simulink model "jacobianComparison"  (R2016a)
settings: Solver=ode4  StartTime=0.0  StopTime=10.0  FixedStep=0.001  RelTol=1e-3
libraries: lwr_dynamics x2
settings Model: Creator=shahriari  LastModifiedBy=shahriari

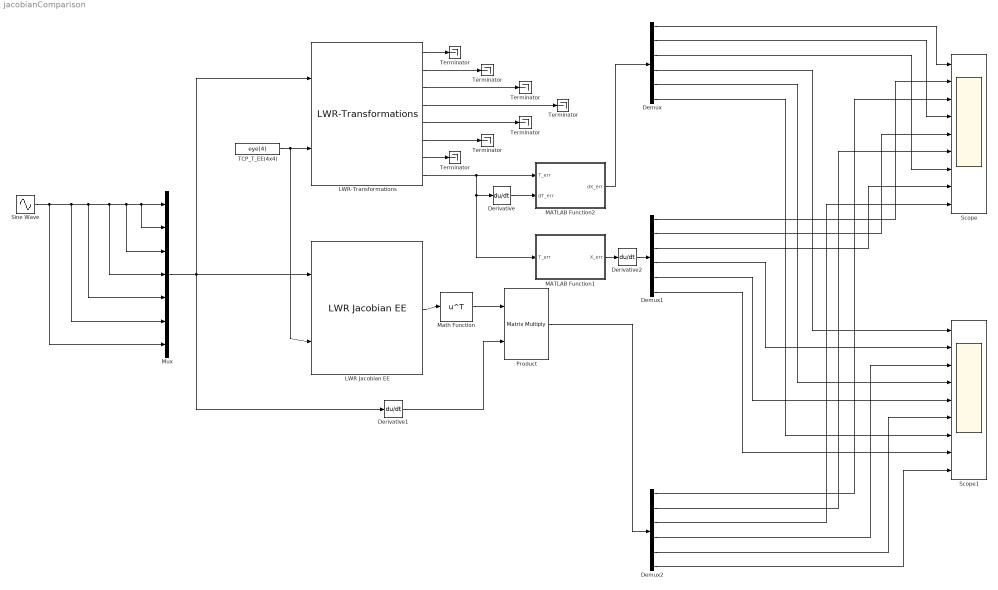
== system jacobianComparison ==
  Demux : Demux  Outputs=6
  Demux1 : Demux  Outputs=6
  Demux2 : Demux  Outputs=6
  Derivative : Derivative
  Derivative1 : Derivative
  Derivative2 : Derivative
  LWR Jacobian EE : lwr_dynamics/Kinematics/LWR Jacobian EE
  LWR-Transformations : lwr_dynamics/Kinematics/LWR-Transformations
  MATLAB Function1 : MATLAB Function  TreatAsAtomicUnit=on
  MATLAB Function2 : MATLAB Function  TreatAsAtomicUnit=on
  Math Function : Math  Operator=transpose  SaturateOnIntegerOverflow=on
  Mux : Mux  Inputs=7
  Product : Product  Multiplication=Matrix(*)
  Scope : Scope  NumInputPorts=9
  Scope1 : Scope  NumInputPorts=9
  Sine Wave : Sin  Bias=0.1  SampleTime=0
  TCP_T_EE(4x4) : Constant  Value=eye(4)
  Terminator : Terminator
  "Terminator " : Terminator
  "Terminator  " : Terminator
  "Terminator   " : Terminator
  "Terminator    " : Terminator
  "Terminator     " : Terminator
  "Terminator      " : Terminator
  wires:
  TCP_T_EE(4x4)/1 -> LWR Jacobian EE/2, LWR-Transformations/2
  Mux/1 -> LWR-Transformations/1, LWR Jacobian EE/1, Derivative1/1
  LWR-Transformations/1 -> Terminator/1
  LWR-Transformations/2 -> "Terminator "/1
  LWR-Transformations/3 -> "Terminator  "/1
  LWR-Transformations/4 -> "Terminator   "/1
  LWR-Transformations/5 -> "Terminator    "/1
  LWR-Transformations/6 -> "Terminator     "/1
  LWR-Transformations/7 -> "Terminator      "/1
  LWR Jacobian EE/1 -> Math Function/1
  Math Function/1 -> Product/1
  LWR-Transformations/8 -> MATLAB Function1/1(T_err), Derivative/1, MATLAB Function2/1(T_err)
  Derivative/1 -> MATLAB Function2/2(dT_err)
  Derivative1/1 -> Product/2
  MATLAB Function2/1(dX_err) -> Demux/1
  Product/1 -> Demux2/1
  MATLAB Function1/1(X_err) -> Derivative2/1
  Derivative2/1 -> Demux1/1
  Demux/1 -> Scope/1
  Demux/2 -> Scope/4
  Demux/3 -> Scope/7
  Demux1/1 -> Scope/2
  Demux1/2 -> Scope/5
  Demux1/3 -> Scope/8
  Demux2/1 -> Scope/3
  Demux2/2 -> Scope/6
  Demux2/3 -> Scope/9
  Demux/4 -> Scope1/1
  Demux/5 -> Scope1/4
  Demux/6 -> Scope1/7
  Demux1/4 -> Scope1/2
  Demux1/5 -> Scope1/5
  Demux1/6 -> Scope1/8
  Demux2/4 -> Scope1/3
  Demux2/5 -> Scope1/6
  Demux2/6 -> Scope1/9
  Sine Wave/1 -> Mux/7, Mux/6, Mux/5, Mux/4, Mux/3, Mux/2, Mux/1

== matlab function jacobianComparison/MATLAB Function1 ==
  data: T_err input; X_err output
function X_err  = fcn(T_err)
%#codegen

X_err = [T_err(1:3,4);rotm2eul(T_err(1:3,1:3))'];

== matlab function jacobianComparison/MATLAB Function2 ==
  data: T_err input; dX_err output; dT_err input
function dX_err  = fcn(T_err, dT_err)
%#codegen

R_err = T_err(1:3,1:3);
dR_err = dT_err(1:3,1:3);
dP_err = dT_err(1:3,4);
omega_str_err = dR_err*R_err';
dX_err = [dP_err;-omega_str_err(2,3);omega_str_err(1,3);-omega_str_err(1,2)];
